simulink model "SF103A_MotRefMdl"  (R2013b)
settings: Solver=FixedStepDiscrete  StartTime=0.0  StopTime=2  FixedStep=.002  RelTol=1e-3
values from neighbouring files (symbols this model uses):
  ARCHGLBPRM_2MILLISEC_SEC_F32 = DataDict.Constant    [SF103A_MotRefMdl_DataDict.m]
  ARCHGLBPRM_2OVERSQRT3_ULS_F32 = DataDict.Constant    [SF103A_MotRefMdl_DataDict.m]
  ARCHGLBPRM_2PI_ULS_F32 = DataDict.Constant    [SF103A_MotRefMdl_DataDict.m]
  ARCHGLBPRM_4OVERSQRT3_ULS_F32 = DataDict.Constant    [SF103A_MotRefMdl_DataDict.m]
  ARCHGLBPRM_5PIOVER4_ULS_F32 = DataDict.Constant    [SF103A_MotRefMdl_DataDict.m]
  ARCHGLBPRM_FLOATZEROTHD_ULS_F32 = DataDict.Constant    [SF103A_MotRefMdl_DataDict.m]
  ARCHGLBPRM_HALFSQRT3_ULS_F32 = DataDict.Constant    [SF103A_MotRefMdl_DataDict.m]
  ARCHGLBPRM_PI_ULS_F32 = DataDict.Constant    [SF103A_MotRefMdl_DataDict.m]
  MotRefMdlCurrDaxBoostGain = DataDict.Calibration    [SF103A_MotRefMdl_DataDict.m]
  MotRefMdlCurrDaxQaxRefDelta = DataDict.Calibration    [SF103A_MotRefMdl_DataDict.m]
  MotRefMdlCurrItrnTolr = DataDict.Calibration    [SF103A_MotRefMdl_DataDict.m]
  MotRefMdlFbCtrlDi = DataDict.Calibration    [SF103A_MotRefMdl_DataDict.m]
  MotRefMdlIvtrDeadTiBrdgVltgSca = DataDict.Calibration    [SF103A_MotRefMdl_DataDict.m]
  MotRefMdlMinCurrItrnLim = DataDict.Calibration    [SF103A_MotRefMdl_DataDict.m]
  MotRefMdlMotCurrDaxMaxSca = DataDict.Calibration    [SF103A_MotRefMdl_DataDict.m]
  MotRefMdlMotVltgDerivtvTiCon = DataDict.Calibration    [SF103A_MotRefMdl_DataDict.m]
  MotRefMdlRefLocnItrnLim = DataDict.Calibration    [SF103A_MotRefMdl_DataDict.m]
  MotRefMdlTqItrnLim = DataDict.Calibration    [SF103A_MotRefMdl_DataDict.m]
  MotRefMdlTqItrnTolr = DataDict.Calibration    [SF103A_MotRefMdl_DataDict.m]
  MotRefMdlVltgModDynCmpEna = DataDict.Calibration    [SF103A_MotRefMdl_DataDict.m]
  MotRefMdlVltgOverRThdSca = DataDict.Calibration    [SF103A_MotRefMdl_DataDict.m]
  SysGlbPrmMotPoleCnt = DataDict.ImprtdCal    [SF103A_MotRefMdl_DataDict.m]
undefined symbols (not defined in the file or in its folder): MotQuad1
libraries: NxtrLim x18, simulink x4, LnrIntrpn x3, Fil x2, NxtrAbslt x2, FixdToFloat x2, FloatToFixd x2, NxtrMath x1
(part 2 of 7)

== system SF103A_MotRefMdl/MotRefMdl/MotRefMdlPer1/ApplyTorqueLimit ==
  note: pass-thru blocks
  MotTqCmd : Inport  RequirementInfo={} %GIDa_025c6779_9066_4c26_ac7c_c60ce040d302
  PeakTq : Inport  RequirementInfo={} %GIDa_b2cef569_5ac6_4023_b455_5bd3826089a9  Port=2
  Abs : Abs  RequirementInfo="{'linktype_rmi_doors' '0000bb42 (/E-STEER Core/SubSystem Specifications/Application Functions/SF99/SF103A Motor Reference Model)' '#SF103A_102' 'true' 'REQ:  SF103A_102' '' } %GIDa_0a8c4a31_5582_4ed5_a511_fc446f1c3802"
  Abs1 : Abs  RequirementInfo="{'linktype_rmi_doors' '0000bb42 (/E-STEER Core/SubSystem Specifications/Application Functions/SF99/SF103A Motor Reference Model)' '#SF103A_102' 'true' 'REQ:  SF103A_102' '' } %GIDa_2b7d6e19_285c_4413_8db0_5b71cefe1f49"
  CopyRight2 : Subsystem  Description=|  mask(Copyright Information){none=on}
      | Copyright info block.                                               
      |                                                                     
      | Place copyright information at the top of every subsystem in design.
      mask prompts: none "No parameters"
      mask help: Place copyright information at the top of every subsystem in design.
      mask Display:
      | NxtrConf = 'Nexteer Confidential';
      | 
      | sys = bdroot; %handle for the current model ("system")
      | first = get_param(sys,'Created');
      | first = first(end-3:end);  %year is last four digits
      | 
      | last = get_param(sys,'LastModifiedDate');
      | if isempty(last)
      |     last = datestr(now,'yyyy');
      | else
      |     last = last(end-3:end);
      | end
      | 
      | if strcmp(first,last)
      |     fprintf('%s -- Copyright %s Nexteer',NxtrConf,first)
      | else
      |     fprintf('%s -- %s%s- %s Nexteer',NxtrConf,char(169),first,last)
      | end
  DisplayVar : DataStoreWrite  DataStoreName=dMotRefMdlMotTqCmdLimd
  If : If  RequirementInfo="{'linktype_rmi_doors' '0000bb42 (/E-STEER Core/SubSystem Specifications/Application Functions/SF99/SF103A Motor Reference Model)' '#SF103A_102' 'true' 'REQ:  SF103A_102' '' } %GIDa_f89377aa_d854_4d40_a11f_6bbea04da2f3"  NumInputs=2  IfExpression=u1 < u2
  If Action Subsystem : Subsystem  RequirementInfo="{'linktype_rmi_doors' '0000bb42 (/E-STEER Core/SubSystem Specifications/Application Functions/SF99/SF103A Motor Reference Model)' '#SF103A_102' 'true' 'REQ:  SF103A_102' '' } %GIDa_32770edd_4c45_4b2d_99de_6da2954c3238"  TreatAsAtomicUnit=on
  If Action Subsystem1 : Subsystem  RequirementInfo="{'linktype_rmi_doors' '0000bb42 (/E-STEER Core/SubSystem Specifications/Application Functions/SF99/SF103A Motor Reference Model)' '#SF103A_102' 'true' 'REQ:  SF103A_102' '' } %GIDa_7552b223_197d_4ca3_8265_c39c5904183a"  TreatAsAtomicUnit=on
  Merge : Merge  RequirementInfo="{'linktype_rmi_doors' '0000bb42 (/E-STEER Core/SubSystem Specifications/Application Functions/SF99/SF103A Motor Reference Model)' '#SF103A_102' 'true' 'REQ:  SF103A_102' '' } %GIDa_db886489_62db_4718_9827_489e9b249dd2"
  MotTqCmdLimd : Outport  RequirementInfo={} %GIDa_be70fa3d_feb5_4f31_bfcb_09d432719c8e
  wires:
  MotTqCmd/1 -> If Action Subsystem/1(In1), Abs/1
  PeakTq/1 -> If Action Subsystem1/1(In1), Abs1/1
  Abs/1 -> If/1
  Abs1/1 -> If/2
  If/1 -> If Action Subsystem/Action
  If/2 -> If Action Subsystem1/Action
  If Action Subsystem/1(Out1) -> Merge/1
  If Action Subsystem1/1(Out1) -> Merge/2
  Merge/1 -> DisplayVar/1, MotTqCmdLimd/1

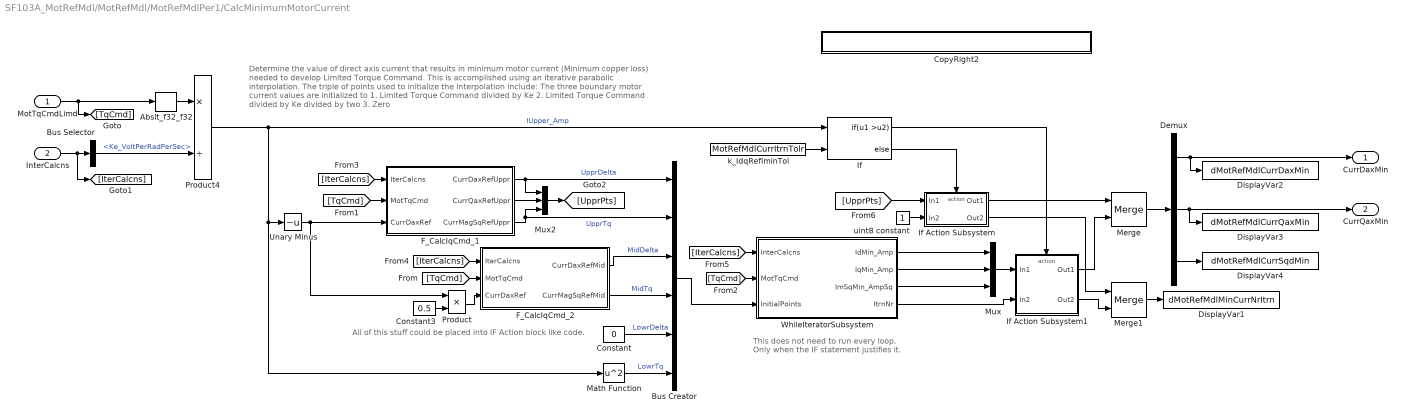
== system SF103A_MotRefMdl/MotRefMdl/MotRefMdlPer1/CalcMinimumMotorCurrent ==
  note: All of this stuff could be placed into IF Action block like code.
  note: Determine the value of direct axis current that results in minimum motor current (Minimum copper loss) needed to develop Limited Torque Command.
      | This is accomplished using an iterative parabolic interpolation. The triple of points used to initialize the interpolation include:
      | The three boundary motor current values are initialized to
      | 1.  Limited Torque Command divided by Ke
      | 2.  Limited Torque Command divided by Ke divided by two
      | 3.  Zero
  note: This does not need to run every loop.
      | Only when the IF statement justifies it.
  MotTqCmdLimd : Inport  RequirementInfo={} %GIDa_27335372_5c13_4910_966a_97541e019b81
  InterCalcns : Inport  RequirementInfo={} %GIDa_5d3d19b5_8e0a_49c0_827d_1a912b33df23  Port=2
  Abslt_f32_f32 : NxtrAbslt/Abslt_f32_f32  RequirementInfo="{'linktype_rmi_doors' '0000bb42 (/E-STEER Core/SubSystem Specifications/Application Functions/SF99/SF103A Motor Reference Model)' '#SF103A_104' 'true' 'REQ:  SF103A_104' '' ; 'linktype_rmi_doors' '0000bb42 (/E-STEER Core/SubSystem Specifications/Application Functions/SF99/SF103A Motor Reference Model)' '#SF103A_105' 'true' 'REQ:  SF103A_105' '' } %GIDa_8dec22c8_c6ec_406f_b8b6_07842b915ec2"  SFunctionSpec=single y1 = Abslt_f32_f32(single u1)
      settings: AttributesFormatString=%<Name>
  Bus Creator : BusCreator  RequirementInfo="{'linktype_rmi_doors' '0000bb42 (/E-STEER Core/SubSystem Specifications/Application Functions/SF99/SF103A Motor Reference Model)' '#SF103A_104' 'true' 'REQ:  SF103A_104' '' } %GIDa_e35f0498_e63d_46c0_a029_eb9455115fce"  Inputs=6
  Bus Selector : BusSelector  RequirementInfo={} %GIDa_044fe998_bec8_4c9c_ae36_7e96b13c3248  OutputSignals=Ke_VoltPerRadPerSec
  Constant : Constant  RequirementInfo="{'linktype_rmi_doors' '0000bb42 (/E-STEER Core/SubSystem Specifications/Application Functions/SF99/SF103A Motor Reference Model)' '#SF103A_104' 'true' 'REQ:  SF103A_104' '' ; 'linktype_rmi_doors' '0000bb42 (/E-STEER Core/SubSystem Specifications/Application Functions/SF99/SF103A Motor Reference Model)' '#SF103A_105' 'true' 'REQ:  SF103A_105' '' } %GIDa_b6256383_66c4_4865_8773_3d52cb1c198c"  Value=0  OutDataTypeStr=single
  Constant3 : Constant  RequirementInfo="{'linktype_rmi_doors' '0000bb42 (/E-STEER Core/SubSystem Specifications/Application Functions/SF99/SF103A Motor Reference Model)' '#SF103A_81' 'true' 'REQ:  SF103A_81' '' ; 'linktype_rmi_doors' '0000bb42 (/E-STEER Core/SubSystem Specifications/Application Functions/SF99/SF103A Motor Reference Model)' '#SF103A_112' 'true' 'REQ:  SF103A_112' '' ; 'linktype_rmi_doors' '0000bb42 (/E-STEER Core/SubSystem Specifications/Application Functions/SF99/SF103A Motor Reference Model)' '#SF103A_104' 'true' 'REQ:  SF103A_104' '' ; 'linktype_rmi_doors' '0000bb42 (/E-STEER Core/SubSystem Specifications/Application Functions/SF99/SF103A Motor Reference Model)' '#SF103A_105' 'true' 'REQ:  SF103A_105' '' } %GIDa_b6152513_7ab6_4c11_a41d_9e137f359da4"  Value=0.5  OutDataTypeStr=single
  CopyRight2 : Subsystem  Description=|  mask(Copyright Information){none=on}
      | Copyright info block.                                               
      |                                                                     
      | Place copyright information at the top of every subsystem in design.
      mask prompts: none "No parameters"
      mask help: Place copyright information at the top of every subsystem in design.
      mask Display:
      | NxtrConf = 'Nexteer Confidential';
      | 
      | sys = bdroot; %handle for the current model ("system")
      | first = get_param(sys,'Created');
      | first = first(end-3:end);  %year is last four digits
      | 
      | last = get_param(sys,'LastModifiedDate');
      | if isempty(last)
      |     last = datestr(now,'yyyy');
      | else
      |     last = last(end-3:end);
      | end
      | 
      | if strcmp(first,last)
      |     fprintf('%s -- Copyright %s Nexteer',NxtrConf,first)
      | else
      |     fprintf('%s -- %s%s- %s Nexteer',NxtrConf,char(169),first,last)
      | end
  Demux : Demux  Outputs=3
  DisplayVar1 : DataStoreWrite  RequirementInfo={} %GIDa_2d0d50f7_8e03_40b7_9215_120c9fd14ca5  DataStoreName=dMotRefMdlMinCurrNrItrn
  DisplayVar2 : DataStoreWrite  DataStoreName=dMotRefMdlCurrDaxMin
  DisplayVar3 : DataStoreWrite  DataStoreName=dMotRefMdlCurrQaxMin
  DisplayVar4 : DataStoreWrite  DataStoreName=dMotRefMdlCurrSqdMin
  F_CalcIqCmd_1 : Subsystem  RequirementInfo="{'linktype_rmi_doors' '0000bb42 (/E-STEER Core/SubSystem Specifications/Application Functions/SF99/SF103A Motor Reference Model)' '#SF103A_104' 'true' 'REQ:  SF103A_104' '' } %GIDa_619eb346_1179_42f5_badf_11c8c11afa26"
  F_CalcIqCmd_2 : Subsystem  RequirementInfo="{'linktype_rmi_doors' '0000bb42 (/E-STEER Core/SubSystem Specifications/Application Functions/SF99/SF103A Motor Reference Model)' '#SF103A_104' 'true' 'REQ:  SF103A_104' '' } %GIDa_a72a8716_719c_4bc9_ac96_f5f0860ac21a"
  If : If  RequirementInfo="{'linktype_rmi_doors' '0000bb42 (/E-STEER Core/SubSystem Specifications/Application Functions/SF99/SF103A Motor Reference Model)' '#SF103A_104' 'true' 'REQ:  SF103A_104' '' } %GIDa_f8ed7dd9_d121_47b1_84c7_a2bc7653a8e5"  NumInputs=2  IfExpression=u1 >u2
  If Action Subsystem : Subsystem  RequirementInfo="{'linktype_rmi_doors' '0000bb42 (/E-STEER Core/SubSystem Specifications/Application Functions/SF99/SF103A Motor Reference Model)' '#SF103A_104' 'true' 'REQ:  SF103A_104' '' } %GIDa_316f97d2_1872_45f5_b3c5_43c5f5a4d490"  TreatAsAtomicUnit=on
      settings: AttributesFormatString=pass_thru
  If Action Subsystem1 : Subsystem  RequirementInfo="{'linktype_rmi_doors' '0000bb42 (/E-STEER Core/SubSystem Specifications/Application Functions/SF99/SF103A Motor Reference Model)' '#SF103A_104' 'true' 'REQ:  SF103A_104' '' } %GIDa_0f41fdb7_f8d5_4528_97fe_9c4fd88b55f1"  TreatAsAtomicUnit=on
  Math Function : Math  RequirementInfo="{'linktype_rmi_doors' '0000bb42 (/E-STEER Core/SubSystem Specifications/Application Functions/SF99/SF103A Motor Reference Model)' '#SF103A_104' 'true' 'REQ:  SF103A_104' '' } %GIDa_25f81ff0_1c73_4788_9413_833cf3a23574"  Operator=square  SaturateOnIntegerOverflow=on
  Merge : Merge  RequirementInfo="{'linktype_rmi_doors' '0000bb42 (/E-STEER Core/SubSystem Specifications/Application Functions/SF99/SF103A Motor Reference Model)' '#SF103A_104' 'true' 'REQ:  SF103A_104' '' } %GIDa_771f4a17_7467_4457_88ef_3aa4770718b3"
  Merge1 : Merge  RequirementInfo="{'linktype_rmi_doors' '0000bb42 (/E-STEER Core/SubSystem Specifications/Application Functions/SF99/SF103A Motor Reference Model)' '#SF103A_104' 'true' 'REQ:  SF103A_104' '' } %GIDa_a7c01730_c045_4cc9_a099_c8b9c00480a4"
  Mux : Mux  RequirementInfo="{'linktype_rmi_doors' '0000bb42 (/E-STEER Core/SubSystem Specifications/Application Functions/SF99/SF103A Motor Reference Model)' '#SF103A_104' 'true' 'REQ:  SF103A_104' '' } %GIDa_375c96f2_0347_495b_ad0e_41acd5e94359"  Inputs=3
  Mux2 : Mux  RequirementInfo={} %GIDa_7b0a7505_f370_4c6e_bc69_7fcf6b8b5241  Inputs=3
  Product : Product  RequirementInfo="{'linktype_rmi_doors' '0000bb42 (/E-STEER Core/SubSystem Specifications/Application Functions/SF99/SF103A Motor Reference Model)' '#SF103A_104' 'true' 'REQ:  SF103A_104' '' ; 'linktype_rmi_doors' '0000bb42 (/E-STEER Core/SubSystem Specifications/Application Functions/SF99/SF103A Motor Reference Model)' '#SF103A_105' 'true' 'REQ:  SF103A_105' '' } %GIDa_54817e69_0090_45e2_a078_cb413413eacf"
  Product4 : Product  RequirementInfo="{'linktype_rmi_doors' '0000bb42 (/E-STEER Core/SubSystem Specifications/Application Functions/SF99/SF103A Motor Reference Model)' '#SF103A_104' 'true' 'REQ:  SF103A_104' '' ; 'linktype_rmi_doors' '0000bb42 (/E-STEER Core/SubSystem Specifications/Application Functions/SF99/SF103A Motor Reference Model)' '#SF103A_105' 'true' 'REQ:  SF103A_105' '' } %GIDa_79fd69e8_2d32_42ff_b268_bdd2d30d6c6f"  Inputs=*/  OutDataTypeStr=Inherit: Inherit via back propagation  RndMeth=Zero
  Unary Minus : UnaryMinus  RequirementInfo="{'linktype_rmi_doors' '0000bb42 (/E-STEER Core/SubSystem Specifications/Application Functions/SF99/SF103A Motor Reference Model)' '#SF103A_104' 'true' 'REQ:  SF103A_104' '' } %GIDa_861a66f3_4944_49a5_b6fb_06229d671546"
  WhileIteratorSubsystem : Subsystem  RequirementInfo="{'linktype_rmi_doors' '0000bb42 (/E-STEER Core/SubSystem Specifications/Application Functions/SF99/SF103A Motor Reference Model)' '#SF103A_104' 'true' 'REQ:  SF103A_104' '' ; 'linktype_rmi_doors' '0000bb42 (/E-STEER Core/SubSystem Specifications/Application Functions/SF99/SF103A Motor Reference Model)' '#SF103A_108' 'true' 'REQ:  SF103A_108' '' } %GIDa_7ae51bf8_618e_4587_91a6_54cdd811713f"  TreatAsAtomicUnit=on
  k_IdqRefIminTol : Constant  RequirementInfo="{'linktype_rmi_doors' '0000bb42 (/E-STEER Core/SubSystem Specifications/Application Functions/SF99/SF103A Motor Reference Model)' '#SF103A_104' 'true' 'REQ:  SF103A_104' '' } %GIDa_f786171e_9c32_4a9c_980a_ca2cd857e056"  Value=MotRefMdlCurrItrnTolr
  uint8 constant : Constant  OutDataTypeStr=uint8
  CurrDaxMin : Outport  RequirementInfo={} %GIDa_40ebe4f4_3f8c_4f1c_94dd_718d4dee145c
  CurrQaxMin : Outport  Port=2
  wires:
  Demux/2 -> CurrQaxMin/1, DisplayVar3/1
  WhileIteratorSubsystem/2(IqMin_Amp) -> Mux/2
  WhileIteratorSubsystem/1(IdMin_Amp) -> Mux/1
  Demux/3 -> DisplayVar4/1
  Mux/1 -> If Action Subsystem1/1(In1)
  WhileIteratorSubsystem/3(ImSqMin_AmpSq) -> Mux/3
  Bus Creator/1 -> WhileIteratorSubsystem/3(InitialPoints)
  Math Function/1 -> Bus Creator/6  "LowrTq"
  Constant/1 -> Bus Creator/5  "LowrDelta"
  F_CalcIqCmd_2/2(CurrMagSqRefMid) -> Bus Creator/4  "MidTq"
  F_CalcIqCmd_2/1(CurrDaxRefMid) -> Bus Creator/3  "MidDelta"
  Product/1 -> F_CalcIqCmd_2/3("CurrDaxRef ")
  F_CalcIqCmd_1/1(CurrDaxRefUppr) -> Bus Creator/1, Mux2/1  "UpprDelta"
  Unary Minus/1 -> Product/1, F_CalcIqCmd_1/3("CurrDaxRef ")
  MotTqCmdLimd/1 -> Abslt_f32_f32/1, [TqCmd]
  F_CalcIqCmd_1/2(CurrQaxRefUppr) -> Mux2/2
  Bus Selector/1 -> Product4/2  "<Ke_VoltPerRadPerSec>"
  [TqCmd] -> F_CalcIqCmd_2/2(MotTqCmd)
  [TqCmd] -> F_CalcIqCmd_1/2(MotTqCmd)
  [TqCmd] -> WhileIteratorSubsystem/2(MotTqCmd)
  Abslt_f32_f32/1 -> Product4/1
  [IterCalcns] -> F_CalcIqCmd_1/1(IterCalcns)
  [IterCalcns] -> F_CalcIqCmd_2/1(IterCalcns)
  [IterCalcns] -> WhileIteratorSubsystem/1(InterCalcns)
  InterCalcns/1 -> [IterCalcns], Bus Selector/1
  Constant3/1 -> Product/2
  k_IdqRefIminTol/1 -> If/2
  Merge/1 -> Demux/1
  If/1 -> If Action Subsystem1/Action
  [UpprPts] -> If Action Subsystem/1(In1)
  F_CalcIqCmd_1/3(CurrMagSqRefUppr) -> Mux2/3, Bus Creator/2  "UpprTq"
  Mux2/1 -> [UpprPts]
  Product4/1 -> Math Function/1, Unary Minus/1, If/1  "IUpper_Amp"
  If/2 -> If Action Subsystem/Action
  If Action Subsystem/1(Out1) -> Merge/1
  If Action Subsystem1/1(Out1) -> Merge/2
  Demux/1 -> DisplayVar2/1, CurrDaxMin/1
  uint8 constant/1 -> If Action Subsystem/2(In2)
  Merge1/1 -> DisplayVar1/1
  WhileIteratorSubsystem/4(ItrnNr) -> If Action Subsystem1/2(In2)
  If Action Subsystem/2(Out2) -> Merge1/1
  If Action Subsystem1/2(Out2) -> Merge1/2

== system SF103A_MotRefMdl/MotRefMdl/MotRefMdlPer1/CopyRight2 ==

== system SF103A_MotRefMdl/MotRefMdl/MotRefMdlPer1/DAxisCurrentBoost ==
  note: "boost crap"
  note: Calculates an alternate Id min value from the Locate Minimum Motor Current Subfunction and its corresponding Iq value.
      | This is to allow for more gradual Id currrent increase as motor velocity increases for a given Limited Torque Command to
      | prevent sudden changes and/or limit cycles in the computed Id min current.
  note: /**** D axis Current boost****/
  MotTqCmdLimd : Inport  RequirementInfo={} %GIDa_7f298480_7122_460d_aba3_f63274f09e19
  CurrDaxAtPeakTq : Inport  RequirementInfo={} %GIDa_fee028f3_e94b_4f93_88d3_0e22aeed4b9d  Port=2
  InterCalcns : Inport  RequirementInfo={} %GIDa_f087d3e5_a0e1_4001_adad_89fa2a3fd0ea  Port=3
  CurrDaxMin : Inport  RequirementInfo={} %GIDa_58adfb30_7037_4c8c_92e1_1fe39eca1421  Port=4
  CurrQaxMin : Inport  RequirementInfo={} %GIDa_22fab042_4f9f_49b7_afb7_c2938b9f0c91  Port=5
  Boost_Merge : Merge  RequirementInfo="{'linktype_rmi_doors' '0000bb42 (/E-STEER Core/SubSystem Specifications/Application Functions/SF99/SF103A Motor Reference Model)' '#SF103A_147' 'true' 'REQ:  SF103A_147' '' } %GIDa_0055ed7d_5ea0_4a12_bb45_3557696b0147"
  Constant1 : Constant  RequirementInfo="{'linktype_rmi_doors' '0000bb42 (/E-STEER Core/SubSystem Specifications/Application Functions/SF99/SF103A Motor Reference Model)' '#SF103A_147' 'true' 'REQ:  SF103A_147' '' } %GIDa_7ab1acad_c012_4e81_942b_909814222c81"  Value=0  OutDataTypeStr=single
  Constant2 : Constant  RequirementInfo="{'linktype_rmi_doors' '0000bb42 (/E-STEER Core/SubSystem Specifications/Application Functions/SF99/SF103A Motor Reference Model)' '#SF103A_147' 'true' 'REQ:  SF103A_147' '' } %GIDa_9edb3918_9c83_4d75_aff2_9346b8f7a230"  Value=MotRefMdlCurrDaxBoostGain
  CopyRight2 : Subsystem  Description=|  mask(Copyright Information){none=on}
      | Copyright info block.                                               
      |                                                                     
      | Place copyright information at the top of every subsystem in design.
      mask prompts: none "No parameters"
      mask help: Place copyright information at the top of every subsystem in design.
      mask Display:
      | NxtrConf = 'Nexteer Confidential';
      | 
      | sys = bdroot; %handle for the current model ("system")
      | first = get_param(sys,'Created');
      | first = first(end-3:end);  %year is last four digits
      | 
      | last = get_param(sys,'LastModifiedDate');
      | if isempty(last)
      |     last = datestr(now,'yyyy');
      | else
      |     last = last(end-3:end);
      | end
      | 
      | if strcmp(first,last)
      |     fprintf('%s -- Copyright %s Nexteer',NxtrConf,first)
      | else
      |     fprintf('%s -- %s%s- %s Nexteer',NxtrConf,char(169),first,last)
      | end
  Dax_Merge : Merge  RequirementInfo="{'linktype_rmi_doors' '0000bb42 (/E-STEER Core/SubSystem Specifications/Application Functions/SF99/SF103A Motor Reference Model)' '#SF103A_147' 'true' 'REQ:  SF103A_147' '' } %GIDa_f870213c_c3db_47d2_8486_bea0c97a9321"
  DisplayVar : DataStoreWrite  DataStoreName=dMotRefMdlMotCurrDaxBoost
  If : If  RequirementInfo="{'linktype_rmi_doors' '0000bb42 (/E-STEER Core/SubSystem Specifications/Application Functions/SF99/SF103A Motor Reference Model)' '#SF103A_147' 'true' 'REQ:  SF103A_147' '' } %GIDa_b99f7b84_dd59_4861_8d48_bfb2f87421e4"
  If Action Subsystem : Subsystem  RequirementInfo="{'linktype_rmi_doors' '0000bb42 (/E-STEER Core/SubSystem Specifications/Application Functions/SF99/SF103A Motor Reference Model)' '#SF103A_147' 'true' 'REQ:  SF103A_147' '' } %GIDa_af405375_7566_4eb7_9430_731a8e076961"  TreatAsAtomicUnit=on
  Qax_Merge : Merge  RequirementInfo="{'linktype_rmi_doors' '0000bb42 (/E-STEER Core/SubSystem Specifications/Application Functions/SF99/SF103A Motor Reference Model)' '#SF103A_147' 'true' 'REQ:  SF103A_147' '' } %GIDa_e5fe2aed_063c_42a9_afa2_986c0226e77e"
  pass_thru : Subsystem  RequirementInfo="{'linktype_rmi_doors' '0000bb42 (/E-STEER Core/SubSystem Specifications/Application Functions/SF99/SF103A Motor Reference Model)' '#SF103A_147' 'true' 'REQ:  SF103A_147' '' } %GIDa_eb7d2bc4_72f9_4d70_be54_b4be77777592"  TreatAsAtomicUnit=on
  CurrDaxBoostd : Outport  RequirementInfo={} %GIDa_b044d620_30d1_423a_9e7a_3aa42901f1e0
  CurrQaxBoostd : Outport  RequirementInfo={} %GIDa_63071d74_5055_4f06_ba25_15c8d917f12c  Port=2
  wires:
  CurrQaxMin/1 -> If Action Subsystem/2(CurrQaxMin), [IqMin]
  InterCalcns/1 -> If Action Subsystem/3(InterCalcns)
  Constant2/1 -> If/1
  CurrDaxMin/1 -> [IdMin], If Action Subsystem/1(CurrDaxMin)
  If/1 -> If Action Subsystem/Action
  MotTqCmdLimd/1 -> If Action Subsystem/4(MotTqCmdLimd)
  CurrDaxAtPeakTq/1 -> If Action Subsystem/5(CurrDaxAtPeakTq)
  If/2 -> pass_thru/Action
  [IdMin] -> pass_thru/1(In1)
  [IqMin] -> pass_thru/2(In2)
  Constant1/1 -> pass_thru/3(In3)
  If Action Subsystem/1(CurrDaxBoostd) -> Dax_Merge/1
  pass_thru/1(Out1) -> Dax_Merge/2
  If Action Subsystem/3(BoostAmnt) -> Boost_Merge/1
  pass_thru/3(Out3) -> Boost_Merge/2
  If Action Subsystem/2(CurrQaxBoostd) -> Qax_Merge/1
  pass_thru/2(Out2) -> Qax_Merge/2
  Dax_Merge/1 -> CurrDaxBoostd/1
  Qax_Merge/1 -> CurrQaxBoostd/1
  Boost_Merge/1 -> DisplayVar/1

== system SF103A_MotRefMdl/MotRefMdl/MotRefMdlPer1/FeedforwardVoltage ==
  note: Code does not separate into two locations.
      | i.e. only one "block".
  note: The Feedforward Voltage subfunction computes and selects which Vd, Vq voltages are passed to SF-105A Current Regulator and Voltage Limiter as the Feedforward Voltages.
      |
      | When in normal operation (i.e., not in LoA mitigation or Degraded Mode), the Current Regulator is active and the Feedforward Voltages represent the Motor BEMF Voltage.  (i.e., Vq = BEMF Voltage, Vd = 0).
      |
      | When in a Degraded Mode where the Current Regulator is disabled, the Feedforward Voltages represent the voltage required to produce the Motor Referecene Currents as defined by an Inverse Motor Model.
      |
      | The Static Feedforward Reference Voltages were computed previously in the Locate Ref subfunction (MtrVoltDaxFFStatic and MtrVoltQaxFFStatic) using a steady state Inverse Motor Model.
      | This subfunction allows for a selectable feature to sum an additional dynamic term to the Static Feedforward Reference Voltages to increase the bandwidth of the feedforward torque control while in Degraded Mode.
      | The Feedforward Voltage Selection subfunction below selects whether or not to add the dynamic term to create the Feedforward Voltages to be used in Degraded Mode.
  MotCurrDaxCmd : Inport
  MotCurrQaxCmd : Inport  Port=2
  MotVltgDaxFfStat : Inport  Port=3
  MotVltgQaxFfStat : Inport  Port=4
  CurrMeasLoaMtgtnEna : Inport  Port=5
  IvtrLoaMtgtnEn : Inport  Port=6
  InterCalcns : Inport  Port=7
  MotInduQaxEstimd : Inport  Port=8
  MotInduDaxEstimd : Inport  Port=9
  CopyRight2 : Subsystem  Description=|  mask(Copyright Information){none=on}
      | Copyright info block.                                               
      |                                                                     
      | Place copyright information at the top of every subsystem in design.
      mask prompts: none "No parameters"
      mask help: Place copyright information at the top of every subsystem in design.
      mask Display:
      | NxtrConf = 'Nexteer Confidential';
      | 
      | sys = bdroot; %handle for the current model ("system")
      | first = get_param(sys,'Created');
      | first = first(end-3:end);  %year is last four digits
      | 
      | last = get_param(sys,'LastModifiedDate');
      | if isempty(last)
      |     last = datestr(now,'yyyy');
      | else
      |     last = last(end-3:end);
      | end
      | 
      | if strcmp(first,last)
      |     fprintf('%s -- Copyright %s Nexteer',NxtrConf,first)
      | else
      |     fprintf('%s -- %s%s- %s Nexteer',NxtrConf,char(169),first,last)
      | end
  DynamicTermCalc : Subsystem
  FeedforwardSelection : Subsystem
  MotVltgDaxFf : Outport
  MotVltgQaxFf : Outport  Port=2
  wires:
  FeedforwardSelection/1(MotVltgDaxFf) -> MotVltgDaxFf/1
  InterCalcns/1 -> FeedforwardSelection/7(InterCalcns)
  MotVltgDaxFfStat/1 -> FeedforwardSelection/1(MotVltgDaxFfStat)
  MotCurrDaxCmd/1 -> DynamicTermCalc/4(MotCurrDaxCmd)
  MotCurrQaxCmd/1 -> DynamicTermCalc/3(MotCurrQaxCmd)
  DynamicTermCalc/1(MotVltgQaxFfDynTerm) -> FeedforwardSelection/5(MotVltgQaxFfDynTerm)
  DynamicTermCalc/2(MotVltgDaxFfDynTerm) -> FeedforwardSelection/6(MotVltgDaxFfDynTerm)
  CurrMeasLoaMtgtnEna/1 -> FeedforwardSelection/3(CurrMeasLoaMtgtnEna)
  MotVltgQaxFfStat/1 -> FeedforwardSelection/2(MotVltgQaxFfStat)
  MotInduDaxEstimd/1 -> DynamicTermCalc/1(EstLd_Henry)
  MotInduQaxEstimd/1 -> DynamicTermCalc/2(EstLq_Henry)
  FeedforwardSelection/2(MotVltgQaxFf) -> MotVltgQaxFf/1
  IvtrLoaMtgtnEn/1 -> FeedforwardSelection/4(IvtrLoaMtgtnEn)

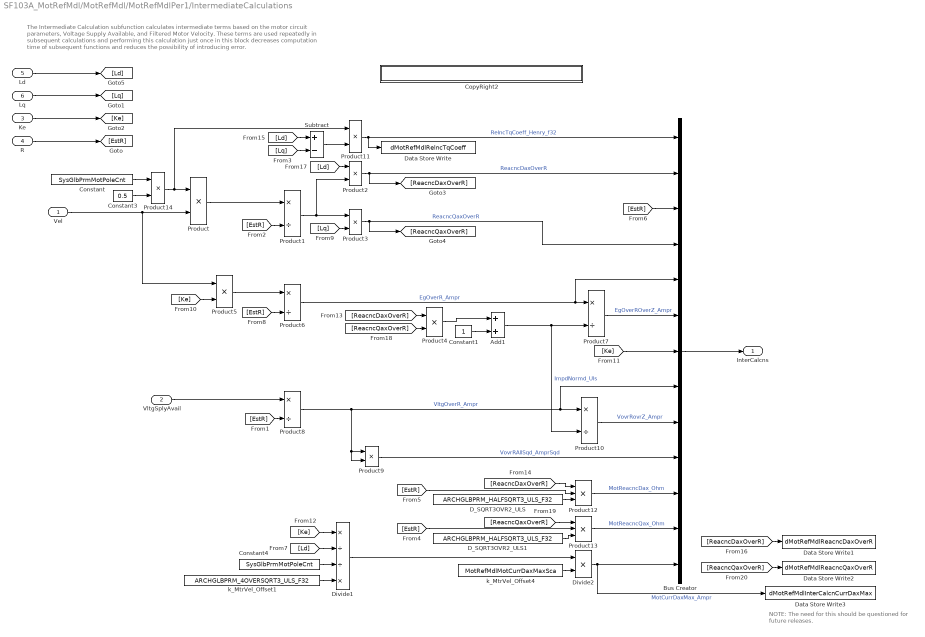
== system SF103A_MotRefMdl/MotRefMdl/MotRefMdlPer1/IntermediateCalculations ==
  note: NOTE:  The need for this should be questioned
      |              for future releases.
  note: The Intermediate Calculation subfunction calculates intermediate terms based on the motor circuit parameters, Voltage Supply Available, and
      | Filtered Motor Velocity.  These terms are used repeatedly in subsequent calculations and performing this calculation just once in this block
      | decreases computation time of subsequent functions and reduces the possibility of introducing error.
  Vel : Inport  RequirementInfo={} %GIDa_2c5d3743_a830_4842_bddc_33849c9eeb79
  VltgSplyAvail : Inport  RequirementInfo={} %GIDa_935be646_aed8_4e40_bb74_4e7aba76f5fc  Port=2
  Ke : Inport  RequirementInfo={} %GIDa_e6d12849_5f91_4425_8566_e61a1afef848  Port=3
  R : Inport  RequirementInfo={} %GIDa_ddce00fe_1cab_4cf5_a622_e268a348c0d3  Port=4
  Ld : Inport  RequirementInfo={} %GIDa_b81a79af_8f4a_4205_b9f0_9b215f46eadd  Port=5
  Lq : Inport  RequirementInfo={} %GIDa_777413d6_8473_4a88_9dad_fcbb9565dc31  Port=6
  Add1 : Sum  RequirementInfo="{'linktype_rmi_doors' '0000bb42 (/E-STEER Core/SubSystem Specifications/Application Functions/SF99/SF103A Motor Reference Model)' '#SF103A_86' 'true' 'REQ:  SF103A_86' '' } %GIDa_8db673c8_96be_4e57_9d72_6795223aa01a"
  Bus Creator : BusCreator  Inputs=13
  Constant : Constant  RequirementInfo="{'linktype_rmi_doors' '0000bb42 (/E-STEER Core/SubSystem Specifications/Application Functions/SF99/SF103A Motor Reference Model)' '#SF103A_80' 'true' 'REQ:  SF103A_80' '' ; 'linktype_rmi_doors' '0000bb42 (/E-STEER Core/SubSystem Specifications/Application Functions/SF99/SF103A Motor Reference Model)' '#SF103A_81' 'true' 'REQ:  SF103A_81' '' ; 'linktype_rmi_doors' '0000bb42 (/E-STEER Core/SubSystem Specifications/Application Functions/SF99/SF103A Motor Reference Model)' '#SF103A_112' 'true' 'REQ:  SF103A_112' '' } %GIDa_0787546e_b3bc_4e61_b6ca_cdea52ef0817"  Value=SysGlbPrmMotPoleCnt
  Constant1 : Constant  RequirementInfo="{'linktype_rmi_doors' '0000bb42 (/E-STEER Core/SubSystem Specifications/Application Functions/SF99/SF103A Motor Reference Model)' '#SF103A_86' 'true' 'REQ:  SF103A_86' '' } %GIDa_f3cac06d_b9f2_48d8_b3bd_472916494482"  OutDataTypeStr=single
  Constant3 : Constant  RequirementInfo="{'linktype_rmi_doors' '0000bb42 (/E-STEER Core/SubSystem Specifications/Application Functions/SF99/SF103A Motor Reference Model)' '#SF103A_81' 'true' 'REQ:  SF103A_81' '' ; 'linktype_rmi_doors' '0000bb42 (/E-STEER Core/SubSystem Specifications/Application Functions/SF99/SF103A Motor Reference Model)' '#SF103A_112' 'true' 'REQ:  SF103A_112' '' } %GIDa_74e2442c_7b8b_4a2d_b0c7_c361dc17b6b1"  Value=0.5  OutDataTypeStr=single
  Constant4 : Constant  RequirementInfo="{'linktype_rmi_doors' '0000bb42 (/E-STEER Core/SubSystem Specifications/Application Functions/SF99/SF103A Motor Reference Model)' '#SF103A_111' 'true' 'REQ:  SF103A_111' '' } %GIDa_7f77aea0_3854_4f0b_b989_a2e29550d679"  Value=SysGlbPrmMotPoleCnt
  CopyRight2 : Subsystem  Description=|  mask(Copyright Information){none=on}
      | Copyright info block.                                               
      |                                                                     
      | Place copyright information at the top of every subsystem in design.
      mask prompts: none "No parameters"
      mask help: Place copyright information at the top of every subsystem in design.
      mask Display:
      | NxtrConf = 'Nexteer Confidential';
      | 
      | sys = bdroot; %handle for the current model ("system")
      | first = get_param(sys,'Created');
      | first = first(end-3:end);  %year is last four digits
      | 
      | last = get_param(sys,'LastModifiedDate');
      | if isempty(last)
      |     last = datestr(now,'yyyy');
      | else
      |     last = last(end-3:end);
      | end
      | 
      | if strcmp(first,last)
      |     fprintf('%s -- Copyright %s Nexteer',NxtrConf,first)
      | else
      |     fprintf('%s -- %s%s- %s Nexteer',NxtrConf,char(169),first,last)
      | end
  D_SQRT3OVR2_ULS : Constant  RequirementInfo="{'linktype_rmi_doors' '0000bb42 (/E-STEER Core/SubSystem Specifications/Application Functions/SF99/SF103A Motor Reference Model)' '#SF103A_113' 'true' 'REQ:  SF103A_113' '' } %GIDa_a4e1215f_7638_4165_aed9_bb274e87cab7"  Value=ARCHGLBPRM_HALFSQRT3_ULS_F32  SampleTime=-1
  D_SQRT3OVR2_ULS1 : Constant  RequirementInfo="{'linktype_rmi_doors' '0000bb42 (/E-STEER Core/SubSystem Specifications/Application Functions/SF99/SF103A Motor Reference Model)' '#SF103A_113' 'true' 'REQ:  SF103A_113' '' } %GIDa_9afad2da_32a0_4aa2_919d_02f88de49dce"  Value=ARCHGLBPRM_HALFSQRT3_ULS_F32  SampleTime=-1
  Data Store Write : DataStoreWrite  DataStoreName=dMotRefMdlRelncTqCoeff
  Data Store Write1 : DataStoreWrite  DataStoreName=dMotRefMdlReacncDaxOverR
  Data Store Write2 : DataStoreWrite  DataStoreName=dMotRefMdlReacncQaxOverR
  Data Store Write3 : DataStoreWrite  DataStoreName=dMotRefMdlInterCalcnCurrDaxMax
  Divide1 : Product  RequirementInfo="{'linktype_rmi_doors' '0000bb42 (/E-STEER Core/SubSystem Specifications/Application Functions/SF99/SF103A Motor Reference Model)' '#SF103A_111' 'true' 'REQ:  SF103A_111' '' } %GIDa_11e7fceb_3fad_4cea_a005_3fdfb2b2a49a"  Inputs=*//*
  Divide2 : Product  RequirementInfo="{'linktype_rmi_doors' '0000bb42 (/E-STEER Core/SubSystem Specifications/Application Functions/SF99/SF103A Motor Reference Model)' '#SF103A_111' 'true' 'REQ:  SF103A_111' '' } %GIDa_a43de061_9dd0_4954_af7a_06b573662fa5"
  Product : Product  RequirementInfo="{'linktype_rmi_doors' '0000bb42 (/E-STEER Core/SubSystem Specifications/Application Functions/SF99/SF103A Motor Reference Model)' '#SF103A_112' 'true' 'REQ:  SF103A_112' '' } %GIDa_73fd4fc6_b2c4_4714_aaec_fb73905af525"  RndMeth=Zero
  Product1 : Product  RequirementInfo="{'linktype_rmi_doors' '0000bb42 (/E-STEER Core/SubSystem Specifications/Application Functions/SF99/SF103A Motor Reference Model)' '#SF103A_112' 'true' 'REQ:  SF103A_112' '' } %GIDa_9f37c5a1_a073_4537_978b_73ac7345120a"  Inputs=*/  RndMeth=Zero
  Product10 : Product  RequirementInfo="{'linktype_rmi_doors' '0000bb42 (/E-STEER Core/SubSystem Specifications/Application Functions/SF99/SF103A Motor Reference Model)' '#SF103A_89' 'true' 'REQ:  SF103A_89' '' } %GIDa_c30c4688_4305_49c8_afcc_e1d3126b3793"  Inputs=*/  RndMeth=Zero
  Product11 : Product  RequirementInfo="{'linktype_rmi_doors' '0000bb42 (/E-STEER Core/SubSystem Specifications/Application Functions/SF99/SF103A Motor Reference Model)' '#SF103A_81' 'true' 'REQ:  SF103A_81' '' } %GIDa_0a02da02_251a_41f2_902b_3e79c1854034"  RndMeth=Zero
  Product12 : Product  RequirementInfo="{'linktype_rmi_doors' '0000bb42 (/E-STEER Core/SubSystem Specifications/Application Functions/SF99/SF103A Motor Reference Model)' '#SF103A_113' 'true' 'REQ:  SF103A_113' '' } %GIDa_14106c50_a189_4040_a6d7_5f4de701bb04"  Inputs=3  RndMeth=Zero
  Product13 : Product  RequirementInfo="{'linktype_rmi_doors' '0000bb42 (/E-STEER Core/SubSystem Specifications/Application Functions/SF99/SF103A Motor Reference Model)' '#SF103A_113' 'true' 'REQ:  SF103A_113' '' } %GIDa_e84c7a76_294b_4b64_97ff_c6a0aff946a0"  Inputs=3  RndMeth=Zero
  Product14 : Product  RequirementInfo="{'linktype_rmi_doors' '0000bb42 (/E-STEER Core/SubSystem Specifications/Application Functions/SF99/SF103A Motor Reference Model)' '#SF103A_81' 'true' 'REQ:  SF103A_81' '' ; 'linktype_rmi_doors' '0000bb42 (/E-STEER Core/SubSystem Specifications/Application Functions/SF99/SF103A Motor Reference Model)' '#SF103A_112' 'true' 'REQ:  SF103A_112' '' } %GIDa_34e56ca3_d24b_4c0b_9ae6_1a69b16f98b8"  RndMeth=Zero
  Product2 : Product  RequirementInfo="{'linktype_rmi_doors' '0000bb42 (/E-STEER Core/SubSystem Specifications/Application Functions/SF99/SF103A Motor Reference Model)' '#SF103A_112' 'true' 'REQ:  SF103A_112' '' } %GIDa_6155009c_eca5_448f_b3f6_92a3b664c0e8"  RndMeth=Zero
  Product3 : Product  RequirementInfo="{'linktype_rmi_doors' '0000bb42 (/E-STEER Core/SubSystem Specifications/Application Functions/SF99/SF103A Motor Reference Model)' '#SF103A_112' 'true' 'REQ:  SF103A_112' '' } %GIDa_3fe8106a_8d80_48e3_9ea6_0e23b09fb3ea"  RndMeth=Zero
  Product4 : Product  RequirementInfo="{'linktype_rmi_doors' '0000bb42 (/E-STEER Core/SubSystem Specifications/Application Functions/SF99/SF103A Motor Reference Model)' '#SF103A_86' 'true' 'REQ:  SF103A_86' '' } %GIDa_eacb5eb3_e032_4667_95c8_ca1e7ba81f7f"  RndMeth=Zero
  Product5 : Product  RequirementInfo="{'linktype_rmi_doors' '0000bb42 (/E-STEER Core/SubSystem Specifications/Application Functions/SF99/SF103A Motor Reference Model)' '#SF103A_85' 'true' 'REQ:  SF103A_85' '' } %GIDa_1510e2f8_2f84_4d52_a5a6_a17cf7701181"  RndMeth=Zero
  Product6 : Product  RequirementInfo="{'linktype_rmi_doors' '0000bb42 (/E-STEER Core/SubSystem Specifications/Application Functions/SF99/SF103A Motor Reference Model)' '#SF103A_85' 'true' 'REQ:  SF103A_85' '' } %GIDa_2f93ed20_bd30_4f24_be8c_ca5775e2697b"  Inputs=*/  RndMeth=Zero
  Product7 : Product  RequirementInfo="{'linktype_rmi_doors' '0000bb42 (/E-STEER Core/SubSystem Specifications/Application Functions/SF99/SF103A Motor Reference Model)' '#SF103A_87' 'true' 'REQ:  SF103A_87' '' } %GIDa_264fb4a3_d399_4c49_830d_762445ca1942"  Inputs=*/  RndMeth=Zero
  Product8 : Product  RequirementInfo="{'linktype_rmi_doors' '0000bb42 (/E-STEER Core/SubSystem Specifications/Application Functions/SF99/SF103A Motor Reference Model)' '#SF103A_88' 'true' 'REQ:  SF103A_88' '' } %GIDa_798b6c50_71d1_49c3_b36a_cecf897886cb"  Inputs=*/  RndMeth=Zero
  Product9 : Product  RequirementInfo="{'linktype_rmi_doors' '0000bb42 (/E-STEER Core/SubSystem Specifications/Application Functions/SF99/SF103A Motor Reference Model)' '#SF103A_88' 'true' 'REQ:  SF103A_88' '' } %GIDa_c59338a3_f7cf_4eb5_b1a5_5be28167d0f1"  RndMeth=Zero
  Subtract : Sum  RequirementInfo="{'linktype_rmi_doors' '0000bb42 (/E-STEER Core/SubSystem Specifications/Application Functions/SF99/SF103A Motor Reference Model)' '#SF103A_81' 'true' 'REQ:  SF103A_81' '' } %GIDa_d9f7810f_1812_4081_aaf9_210e24007ff6"  Inputs=+-
  k_MtrVel_Offset1 : Constant  RequirementInfo="{'linktype_rmi_doors' '0000bb42 (/E-STEER Core/SubSystem Specifications/Application Functions/SF99/SF103A Motor Reference Model)' '#SF103A_111' 'true' 'REQ:  SF103A_111' '' } %GIDa_d4d36dbb_1f33_4dee_b45f_ff6bba25e6ee"  Value=ARCHGLBPRM_4OVERSQRT3_ULS_F32  SampleTime=-1
  k_MtrVel_Offset4 : Constant  RequirementInfo="{'linktype_rmi_doors' '0000bb42 (/E-STEER Core/SubSystem Specifications/Application Functions/SF99/SF103A Motor Reference Model)' '#SF103A_111' 'true' 'REQ:  SF103A_111' '' } %GIDa_a0c68ee5_0180_4ba9_a948_cb4309ae0e8a"  Value=MotRefMdlMotCurrDaxMaxSca  SampleTime=-1
  InterCalcns : Outport
  wires:
  VltgSplyAvail/1 -> Product8/1
  Bus Creator/1 -> InterCalcns/1
  Product10/1 -> Bus Creator/9  "VovrRovrZ_Ampr"
  Product11/1 -> Bus Creator/1, Data Store Write/1  "RelncTqCoeff_Henry_f32"
  [EstR] -> Bus Creator/3
  Product9/1 -> Bus Creator/10  "VovrRAllSqd_AmprSqd"
  Product8/1 -> Product9/2, Product9/1, Product10/1, Bus Creator/8  "VltgOverR_Ampr"
  [EstR] -> Product8/2
  Product7/1 -> Bus Creator/6  "EgOverROverZ_Ampr"
  Product6/1 -> Bus Creator/5, Product7/1  "EgOverR_Ampr"
  [EstR] -> Product1/2
  R/1 -> [EstR]
  Product5/1 -> Product6/1
  [Ke] -> Product5/2
  Add1/1 -> Product7/2, Product10/2  "ImpdNormd_Uls"
  Constant1/1 -> Add1/2
  Product4/1 -> Add1/1
  Lq/1 -> [Lq]
  [Ld] -> Product2/1
  Product1/1 -> Product3/1, Product2/2
  Product/1 -> Product1/1
  Vel/1 -> Product5/1, Product/2
  Product14/1 -> Product11/1, Product/1
  Product3/1 -> Bus Creator/4, [ReacncQaxOverR]  "ReacncQaxOverR"
  [EstR] -> Product13/2
  Product13/1 -> Bus Creator/12  "MotReacncQax_Ohm"
  Product12/1 -> Bus Creator/11  "MotReacncDax_Ohm"
  Product2/1 -> Bus Creator/2, [ReacncDaxOverR]  "ReacncDaxOverR"
  Constant4/1 -> Divide1/3
  Divide1/1 -> Divide2/1
  k_MtrVel_Offset4/1 -> Divide2/2
  Divide2/1 -> Bus Creator/13, Data Store Write3/1  "MotCurrDaxMax_Ampr"
  [Ld] -> Divide1/2
  Constant/1 -> Product14/1
  Constant3/1 -> Product14/2
  [EstR] -> Product12/2
  [EstR] -> Product6/2
  [Lq] -> Product3/2
  Ke/1 -> [Ke]
  [Ke] -> Divide1/1
  k_MtrVel_Offset1/1 -> Divide1/4
  [Lq] -> Subtract/2
  Subtract/1 -> Product11/2
  D_SQRT3OVR2_ULS/1 -> Product12/3
  D_SQRT3OVR2_ULS1/1 -> Product13/3
  [ReacncDaxOverR] -> Product4/1
  [ReacncDaxOverR] -> Product12/1
  [ReacncDaxOverR] -> Data Store Write1/1
  [ReacncQaxOverR] -> Product4/2
  [ReacncQaxOverR] -> Product13/1
  [ReacncQaxOverR] -> Data Store Write2/1
  Ld/1 -> [Ld]
  [Ld] -> Subtract/1
  [Ke] -> Bus Creator/7

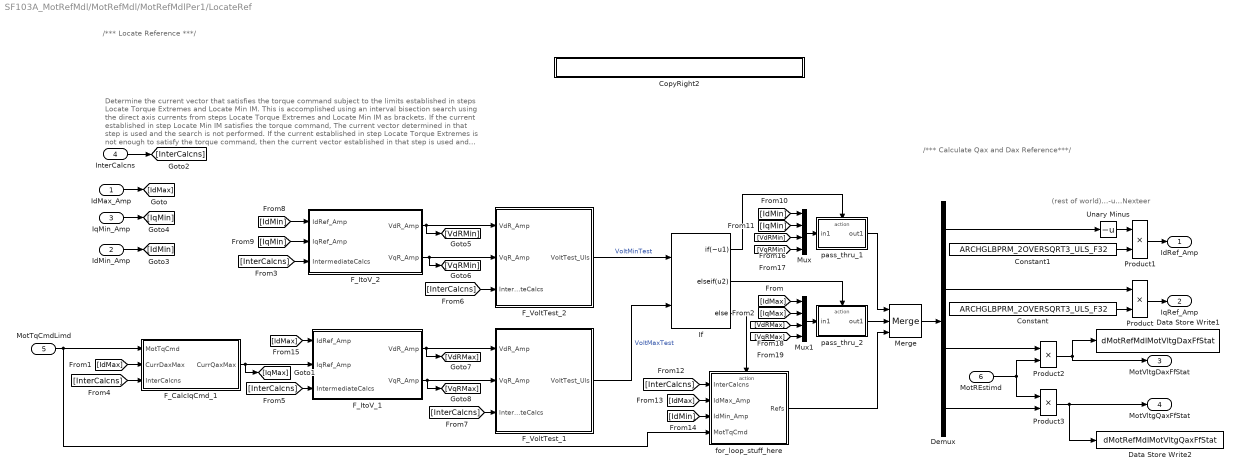
== system SF103A_MotRefMdl/MotRefMdl/MotRefMdlPer1/LocateRef ==
  note: (rest of world)...-u...Nexteer
  note: /*** Calculate Qax and Dax Reference***/
  note: /*** Locate Reference ***/
  note: Determine the current vector that satisfies the torque command subject to the limits established in steps Locate Torque
      | Extremes and Locate Min IM.
      | This is accomplished using an interval bisection search using the direct axis currents from steps Locate Torque Extremes
      | and Locate Min IM as brackets. If the current established in step Locate Min IM satisfies the torque command, The current
      | vector determined in that step is used and the search is not performed. If the current established in step Locate Torque
      | Extremes is not enough to satisfy the torque command, then the current vector established in that step is used and the search
      | is not performed. In all cases, the equations used in establishing the brackets and within the search loop yield the current
      | vector in Cartesian coordinates and also the voltage vector in Cartesian coordinates as an intermediate result.
  IdMax_Amp : Inport
  IdMin_Amp : Inport  RequirementInfo={} %GIDa_0137582e_d1ae_4cf2_b844_3e689d1683d7  Port=2
  IqMin_Amp : Inport  RequirementInfo={} %GIDa_de87edc6_e482_44e6_8481_ad2faa017f2f  Port=3
  InterCalcns : Inport  Port=4
  MotTqCmdLimd : Inport  Port=5
  MotREstimd : Inport  RequirementInfo="{'linktype_rmi_doors' '0000bb42 (/E-STEER Core/SubSystem Specifications/Application Functions/SF99/SF103A Motor Reference Model)' '#SF103A_129' 'true' 'REQ:  SF103A_129' '' } %GIDa_7bb381f7_06df_4bc8_a948_f1ec0b73170c"  Port=6
  Constant : Constant  RequirementInfo="{'linktype_rmi_doors' '0000bb42 (/E-STEER Core/SubSystem Specifications/Application Functions/SF99/SF103A Motor Reference Model)' '#SF103A_128' 'true' 'REQ:  SF103A_128' '' } %GIDa_737e22c8_57a4_4272_95bd_7b97de9fd4e9"  Value=ARCHGLBPRM_2OVERSQRT3_ULS_F32
  Constant1 : Constant  RequirementInfo="{'linktype_rmi_doors' '0000bb42 (/E-STEER Core/SubSystem Specifications/Application Functions/SF99/SF103A Motor Reference Model)' '#SF103A_128' 'true' 'REQ:  SF103A_128' '' } %GIDa_12779e80_1190_4826_af52_7dc96c0ac450"  Value=ARCHGLBPRM_2OVERSQRT3_ULS_F32
  CopyRight2 : Subsystem  Description=|  mask(Copyright Information){none=on}
      | Copyright info block.                                               
      |                                                                     
      | Place copyright information at the top of every subsystem in design.
      mask prompts: none "No parameters"
      mask help: Place copyright information at the top of every subsystem in design.
      mask Display:
      | NxtrConf = 'Nexteer Confidential';
      | 
      | sys = bdroot; %handle for the current model ("system")
      | first = get_param(sys,'Created');
      | first = first(end-3:end);  %year is last four digits
      | 
      | last = get_param(sys,'LastModifiedDate');
      | if isempty(last)
      |     last = datestr(now,'yyyy');
      | else
      |     last = last(end-3:end);
      | end
      | 
      | if strcmp(first,last)
      |     fprintf('%s -- Copyright %s Nexteer',NxtrConf,first)
      | else
      |     fprintf('%s -- %s%s- %s Nexteer',NxtrConf,char(169),first,last)
      | end
  Data Store Write1 : DataStoreWrite  DataStoreName=dMotRefMdlMotVltgDaxFfStat
  Data Store Write2 : DataStoreWrite  DataStoreName=dMotRefMdlMotVltgQaxFfStat
  Demux : Demux
  F_CalcIqCmd_1 : Subsystem  RequirementInfo="{'linktype_rmi_doors' '0000bb42 (/E-STEER Core/SubSystem Specifications/Application Functions/SF99/SF103A Motor Reference Model)' '#SF103A_115' 'true' 'REQ:  SF103A_115' '' } %GIDa_48e0f0d9_d204_4757_b876_83c721969a9a"
  "F_ItoV_1 " : Subsystem  RequirementInfo="{'linktype_rmi_doors' '0000bb42 (/E-STEER Core/SubSystem Specifications/Application Functions/SF99/SF103A Motor Reference Model)' '#SF103A_116' 'true' 'REQ:  SF103A_116' '' } %GIDa_3a1d086e_63c1_41d0_9b1b_034da4de0f93"
  F_ItoV_2 : Subsystem  RequirementInfo="{'linktype_rmi_doors' '0000bb42 (/E-STEER Core/SubSystem Specifications/Application Functions/SF99/SF103A Motor Reference Model)' '#SF103A_116' 'true' 'REQ:  SF103A_116' '' } %GIDa_ceea8677_2a51_421d_ad69_2a8758fc9240"
  F_VoltTest_1 : Subsystem  RequirementInfo="{'linktype_rmi_doors' '0000bb42 (/E-STEER Core/SubSystem Specifications/Application Functions/SF99/SF103A Motor Reference Model)' '#SF103A_120' 'true' 'REQ:  SF103A_120' '' ; 'linktype_rmi_doors' '0000bb42 (/E-STEER Core/SubSystem Specifications/Application Functions/SF99/SF103A Motor Reference Model)' '#SF103A_121' 'true' 'REQ:  SF103A_121' '' ; 'linktype_rmi_doors' '0000bb42 (/E-STEER Core/SubSystem Specifications/Application Functions/SF99/SF103A Motor Reference Model)' '#SF103A_125' 'true' 'REQ:  SF103A_125' '' } %GIDa_6ceb6b7b_74b3_419f_ae72_af0c68b56694"
  F_VoltTest_2 : Subsystem  RequirementInfo="{'linktype_rmi_doors' '0000bb42 (/E-STEER Core/SubSystem Specifications/Application Functions/SF99/SF103A Motor Reference Model)' '#SF103A_119' 'true' 'REQ:  SF103A_119' '' } %GIDa_faf2266a_45d6_428b_a43b_188aa54f1b85"
  If : If  RequirementInfo="{'linktype_rmi_doors' '0000bb42 (/E-STEER Core/SubSystem Specifications/Application Functions/SF99/SF103A Motor Reference Model)' '#SF103A_122' 'true' 'REQ:  SF103A_122' '' ; 'linktype_rmi_doors' '0000bb42 (/E-STEER Core/SubSystem Specifications/Application Functions/SF99/SF103A Motor Reference Model)' '#SF103A_120' 'true' 'REQ:  SF103A_120' '' ; 'linktype_rmi_doors' '0000bb42 (/E-STEER Core/SubSystem Specifications/Application Functions/SF99/SF103A Motor Reference Model)' '#SF103A_121' 'true' 'REQ:  SF103A_121' '' ; 'linktype_rmi_doors' '0000bb42 (/E-STEER Core/SubSystem Specifications/Application Functions/SF99/SF103A Motor Reference Model)' '#SF103A_125' 'true' 'REQ:  SF103A_125' '' } %GIDa_30001bae_ed69_4ddc_876e_7b03419bfa12"  NumInputs=2  IfExpression=~u1  ElseIfExpressions=u2
  Merge : Merge  RequirementInfo="{'linktype_rmi_doors' '0000bb42 (/E-STEER Core/SubSystem Specifications/Application Functions/SF99/SF103A Motor Reference Model)' '#SF103A_122' 'true' 'REQ:  SF103A_122' '' ; 'linktype_rmi_doors' '0000bb42 (/E-STEER Core/SubSystem Specifications/Application Functions/SF99/SF103A Motor Reference Model)' '#SF103A_121' 'true' 'REQ:  SF103A_121' '' ; 'linktype_rmi_doors' '0000bb42 (/E-STEER Core/SubSystem Specifications/Application Functions/SF99/SF103A Motor Reference Model)' '#SF103A_125' 'true' 'REQ:  SF103A_125' '' } %GIDa_3ef48b1c_0d0e_42b0_bf9d_c96d28fd4399"  Inputs=3
  Mux : Mux  RequirementInfo={} %GIDa_c96d0d06_6c28_42b9_a5fb_60b8e8d5cc1b
  Mux1 : Mux  RequirementInfo={} %GIDa_5a83f15e_497d_47c5_a951_461e68d29e81
  Product : Product  RequirementInfo="{'linktype_rmi_doors' '0000bb42 (/E-STEER Core/SubSystem Specifications/Application Functions/SF99/SF103A Motor Reference Model)' '#SF103A_128' 'true' 'REQ:  SF103A_128' '' } %GIDa_55f6eca8_6c73_4b22_b371_db96f8a7f5d4"
  Product1 : Product  RequirementInfo="{'linktype_rmi_doors' '0000bb42 (/E-STEER Core/SubSystem Specifications/Application Functions/SF99/SF103A Motor Reference Model)' '#SF103A_128' 'true' 'REQ:  SF103A_128' '' } %GIDa_3860c754_7453_40f3_8030_fef1714f2784"
  Product2 : Product  RequirementInfo="{'linktype_rmi_doors' '0000bb42 (/E-STEER Core/SubSystem Specifications/Application Functions/SF99/SF103A Motor Reference Model)' '#SF103A_129' 'true' 'REQ:  SF103A_129' '' } %GIDa_9afa8c41_478c_41a7_b447_68776a94ee27"
  Product3 : Product  RequirementInfo="{'linktype_rmi_doors' '0000bb42 (/E-STEER Core/SubSystem Specifications/Application Functions/SF99/SF103A Motor Reference Model)' '#SF103A_129' 'true' 'REQ:  SF103A_129' '' } %GIDa_4fab32fa_dd44_4eac_b856_8794aef379e2"
  Unary Minus : UnaryMinus  RequirementInfo="{'linktype_rmi_doors' '0000bb42 (/E-STEER Core/SubSystem Specifications/Application Functions/SF99/SF103A Motor Reference Model)' '#SF103A_128' 'true' 'REQ:  SF103A_128' '' } %GIDa_6194fd40_2e64_43ba_93d2_c70cb43369e2"
  for_loop_stuff_here : Subsystem  RequirementInfo="{'linktype_rmi_doors' '0000bb42 (/E-STEER Core/SubSystem Specifications/Application Functions/SF99/SF103A Motor Reference Model)' '#SF103A_125' 'true' 'REQ:  SF103A_125' '' } %GIDa_a6f754e7_a790_4aff_b87c_2435d62e2654"  TreatAsAtomicUnit=on
  pass_thru_1 : Subsystem  RequirementInfo="{'linktype_rmi_doors' '0000bb42 (/E-STEER Core/SubSystem Specifications/Application Functions/SF99/SF103A Motor Reference Model)' '#SF103A_122' 'true' 'REQ:  SF103A_122' '' } %GIDa_6017094c_4b57_4668_9835_1eb9f3a648b9"  TreatAsAtomicUnit=on
      settings: RTWSystemCode=Inline
  pass_thru_2 : Subsystem  RequirementInfo="{'linktype_rmi_doors' '0000bb42 (/E-STEER Core/SubSystem Specifications/Application Functions/SF99/SF103A Motor Reference Model)' '#SF103A_121' 'true' 'REQ:  SF103A_121' '' } %GIDa_786ce3ae_e2ea_471e_ba7e_0a1c5a672b02"  TreatAsAtomicUnit=on
  IdRef_Amp : Outport  RequirementInfo={} %GIDa_6400efc8_e20f_4d4d_8637_14f70c8a38cd
  IqRef_Amp : Outport  RequirementInfo={} %GIDa_f8e86ff1_19c2_45a7_b8b2_b7d4ae488d38  Port=2
  MotVltgDaxFfStat : Outport  RequirementInfo={} %GIDa_520d3aa3_89a9_4bb0_adb9_79167a26f1a7  Port=3
  MotVltgQaxFfStat : Outport  RequirementInfo={} %GIDa_19255396_72e6_4e3b_aa93_9062ed70d4bd  Port=4
  wires:
  [IqMin] -> F_ItoV_2/2(IqRef_Amp)
  [IdMin] -> F_ItoV_2/1(IdRef_Amp)
  F_VoltTest_2/1(VoltTest_Uls) -> If/1  "VoltMinTest"
  F_ItoV_2/2(VqR_Amp) -> F_VoltTest_2/2(VqR_Amp), [VqRMin]
  F_ItoV_2/1(VdR_Amp) -> F_VoltTest_2/1(VdR_Amp), [VdRMin]
  If/3 -> for_loop_stuff_here/Action
  If/2 -> pass_thru_2/Action
  If/1 -> pass_thru_1/Action
  IdMax_Amp/1 -> [IdMax]
  [IdMax] -> F_CalcIqCmd_1/2(CurrDaxMax)
  F_CalcIqCmd_1/1(CurrQaxMax) -> [IqMax], "F_ItoV_1 "/2(IqRef_Amp)
  "F_ItoV_1 "/1(VdR_Amp) -> [VdRMax], F_VoltTest_1/1(VdR_Amp)
  "F_ItoV_1 "/2(VqR_Amp) -> [VqRMax], F_VoltTest_1/2(VqR_Amp)
  F_VoltTest_1/1(VoltTest_Uls) -> If/2  "VoltMaxTest"
  InterCalcns/1 -> [InterCalcns]
  [InterCalcns] -> F_ItoV_2/3(IntermediateCalcs)
  [InterCalcns] -> F_CalcIqCmd_1/3(InterCalcns)
  [InterCalcns] -> "F_ItoV_1 "/3(IntermediateCalcs)
  [InterCalcns] -> F_VoltTest_2/3(IntermediateCalcs)
  [InterCalcns] -> F_VoltTest_1/3(IntermediateCalcs)
  IdMin_Amp/1 -> [IdMin]
  [InterCalcns] -> for_loop_stuff_here/1(InterCalcns)
  pass_thru_1/1(out1) -> Merge/1
  [IdMax] -> for_loop_stuff_here/2(IdMax_Amp)
  [IdMin] -> for_loop_stuff_here/3(IdMin_Amp)
  MotTqCmdLimd/1 -> F_CalcIqCmd_1/1(MotTqCmd), for_loop_stuff_here/4(MotTqCmd)
  Constant/1 -> Product/2
  Product/1 -> IqRef_Amp/1
  Constant1/1 -> Product1/2
  Product1/1 -> IdRef_Amp/1
  Unary Minus/1 -> Product1/1
  [IdMax] -> "F_ItoV_1 "/1(IdRef_Amp)
  [IdMax] -> Mux1/1
  [IqMax] -> Mux1/2
  Merge/1 -> Demux/1
  pass_thru_2/1(out1) -> Merge/2
  for_loop_stuff_here/1(Refs) -> Merge/3
  [IdMin] -> Mux/1
  [IqMin] -> Mux/2
  [VdRMin] -> Mux/3
  [VqRMin] -> Mux/4
  Mux/1 -> pass_thru_1/1(in1)
  Mux1/1 -> pass_thru_2/1(in1)
  [VdRMax] -> Mux1/3
  [VqRMax] -> Mux1/4
  Demux/2 -> Product/1
  Demux/3 -> Product2/1
  MotREstimd/1 -> Product2/2, Product3/1
  Demux/4 -> Product3/2
  Product2/1 -> MotVltgDaxFfStat/1, Data Store Write1/1
  Product3/1 -> MotVltgQaxFfStat/1, Data Store Write2/1
  IqMin_Amp/1 -> [IqMin]
  Demux/1 -> Unary Minus/1
